simulink model "spaceship_sim_sol_Euler"  (R2023b)
settings: Solver=ode45  StartTime=0.0  StopTime=30  RelTol=1e-3  EnableMultiTasking=on
values from neighbouring files (symbols this model uses):
  Ic = diag([ 1/12*m*H^2+1/4*m*R^2 ; 1/12*m*H^2+1/4*m*R^2 ; 1/2*m*R^2 ])    [spaceship_par_sol.m]
  m = 9600    [par.m]    (also in spaceship_par_sol.m = 12055)
  M_RB = [ m*eye(3) , zeros(3) ; zeros(3) , Ic ]    [spaceship_par_sol.m]
libraries: vrlib x3, simulink_extras x2, sharedtransform x1
Description:
  | Plane Take-Off with HUD Text
  | 
  | This model is a variant of the vrtkoff example that shows also how to display
  | signal values as text in the virtual scene and a simple Head-Up Display (HUD).
  | 
  | The text is sent to the virtual world as Simulink(R) string signal, composed from the numeric
  | input values using the format string (see sprintf for more information) and sent
  | to the 'string' field of the corresponding Text node in the world. Individual lines of
  | the MFString field are separated by the newline character in the format string.
  | 
  | The HUD behavior (maintaining constant relative position between the user and the
  | Text node) is achieved by defining a ProximitySensor that senses user position and
  | orientation as it navigates through the scene and routing this information to the translation
  | and rotation of HUD object - in this case a VRML Transform that contains the Text node.
settings Model: Creator=The MathWorks, Inc.  LastModifiedBy=jerome
settings SolverCC: AlgebraicLoopSolver=TrustRegion
settings DataIOCC: LimitDataPoints=on  SaveFormat=Array  SaveOutput=off  SaveTime=off  ReturnWorkspaceOutputs=off  SignalLoggingName=logsOut
settings OptimizationCC: BlockReduction=off  BooleanDataType=off  ExpressionDepthLimit=2147483647  InitFltsAndDblsToZero=on  LifeSpan=inf
settings DebuggingCC: UnderspecifiedInitializationDetection=Classic  MergeDetectMultiDrivingBlocksExec=none  CheckExecutionContextPreStartOutputMsg=on  SignalResolutionControl=TryResolveAllWithWarning  MultiTaskDSMMsg=warning  MultiTaskCondExecSysMsg=none  FcnCallInpInsideContextMsg=warning  UnconnectedInputMsg=warning  UnconnectedOutputMsg=warning  UnconnectedLineMsg=warning  StateNameClashWarn=warning  SymbolicDimsDataTypeCodeGenerationDiagnostic=none  SFUnexpectedBacktrackingDiag=warning  SFNoUnconditionalDefaultTransitionDiag=warning  SFExecutionAtInitializationDiag=none  ArithmeticOperatorsInVariantConditions=warning
settings HardwareCC: ProdBitPerPointer=32  ProdBitPerSizeT=32  ProdBitPerPtrDiffT=32  ProdLargestAtomicFloat=None  ProdIntDivRoundTo=Undefined  ProdEndianess=Unspecified  ProdWordSize=32  ProdHWDeviceType=32-bit Generic  TargetUnknown=on
settings ModelReferenceCC: UpdateModelReferenceTargets=IfOutOfDate  EnableRefExpFcnMdlSchedulingChecks=on  PropagateSignalLabelsOutOfModel=off
settings SFSimCC: SimUseLocalCustomCode=off  CustomCodeUndefinedFunction=UseInterfaceOnly
settings RTWCC: RTWUseLocalCustomCode=off  DLArmComputeVersion=19.05
settings CodeAppCC: StateflowObjectComments=on
settings GRTTargetCC: TargetFcnLib=ansi_tfl_tmw.mat  TargetLangStandard=C89/C90 (ANSI)  CombineOutputUpdateFcns=off  GRTInterface=on
settings ConfigComp: CovMetricSettings=d  CovSaveCumulativeToWorkspaceVar=on  CovSaveSingleToWorkspaceVar=on  CovExternalEMLEnable=off  CovSFcnEnable=off

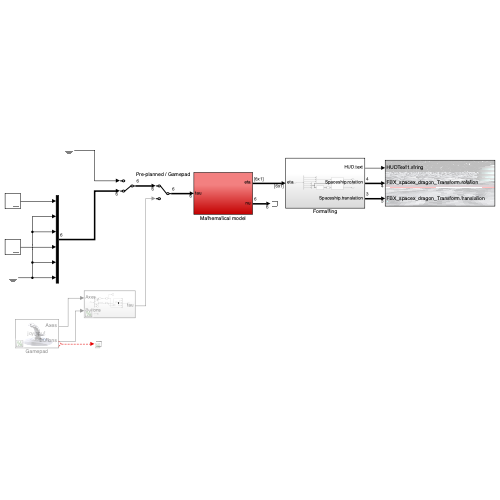
[thumbnail: Simulink's stored preview of the top-level diagram]
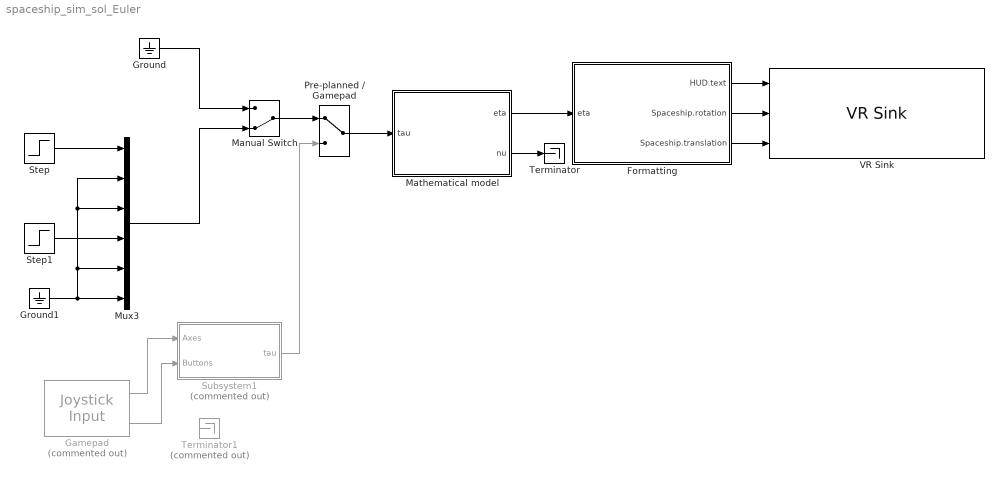
== system spaceship_sim_sol_Euler ==
  Formatting : Subsystem
  Gamepad : vrlib/Joystick Input  Commented=on  joyid=1  adjustports=on  forcefeed=off
  Ground : Ground
  Ground1 : Ground
  Manual Switch : ManualSwitch  CurrentSetting=0
  Mathematical model : Subsystem
  Mux3 : Mux  Inputs=6
  Pre-planned / Gamepad : ManualSwitch
  Step : Step  Before=50000  After=0  SampleTime=0
  Step1 : Step  Before=20000  After=0  SampleTime=0
  Subsystem1 : Subsystem  Commented=on
  Terminator : Terminator
  Terminator1 : Terminator  Commented=on
  VR Sink : vrlib/VR Sink  InstantiateOnLoad=on  SampleTime=0.1  ViewEnable=on  RemoteChange=off  RemoteView=off  FieldsWritten=HUDText1.string.1.-1.1.char#FBX_spacex_dragon_Transform.rotation.4.1.1.double#FBX_spacex_dragon_Transform.translation.3.1.1.double  WorldFileName=spaceship_VR.x3d  WorldDescription=VR Spaceship Dragon  AutoView=off  VideoDimensions=[]  AllowVariableSize=off  FigureProperties="{'Position', 'Name', 'Viewpoint', 'CameraBound', 'CameraDirection', 'CameraPosition', 'CameraUpVector', 'ZoomFactor', 'Antialiasing', 'Headlight', 'Lighting', 'NavPanel', 'Sound', 'StatusBar', 'Stereo3D', 'Stereo3DCameraOffset', 'Stereo3DHIT', 'ToolBar', 'Textures', 'Transparency', 'Triad', 'Wireframe', 'NavZones', 'NavMode', 'NavSpeed', 'CaptureFileFormat', 'CaptureFileName', 'Record2DCompressMethod', 'Record2DCompressQuality', 'Record2D', 'Record2DFileName', 'Record2DFPS'; [5.0000000000000000e+00   1.1600000000000000e+02   5.7600000000000000e+02   3.5000000000000000e+02], 'VR Spaceship Dragon', 'Spaceport', 'on', [0.0000000000000000e+00   0.0000000000000000e+00  -1.0000000000000000e+00], [0.0000000000000000e+00   0.0000000000000000e+00   0.0000000000000000e+00], [0.0000000000000000e+00   1.0000000000000000e+00   0.0000000000000000e+00], [1.0000000000000000e+00], 'on', 'on', 'on', 'halfbar', 'on', 'on', 'off', [1.0000000149011612e-01], [0.0000000000000000e+00], 'on', 'on', 'on', 'none', 'off', 'off', 'fly', 'normal', 'tif', '%f_anim_%n.tif', 'auto', [7.5000000000000000e+01], 'off', '%f_anim_%n.avi', 'auto'}"
  wires:
  Formatting/1(HUD.text) -> VR Sink/1
  Formatting/2(Spaceship.rotation) -> VR Sink/2
  Formatting/3(Spaceship.translation) -> VR Sink/3
  Mathematical model/1(eta) -> Formatting/1(eta)
  Mathematical model/2(nu) -> Terminator/1
  Ground/1 -> Manual Switch/1
  Mux3/1 -> Manual Switch/2
  Ground1/1 -> Mux3/6, Mux3/2, Mux3/3, Mux3/5
  Pre-planned / Gamepad/1 -> Mathematical model/1(tau)
  Manual Switch/1 -> Pre-planned / Gamepad/1
  Gamepad/1 -> Subsystem1/1(Axes)
  Subsystem1/1(tau) -> Pre-planned / Gamepad/2
  Gamepad/2 -> Subsystem1/2(Buttons)
  ? -> Terminator1/1
  Step/1 -> Mux3/1
  Step1/1 -> Mux3/4

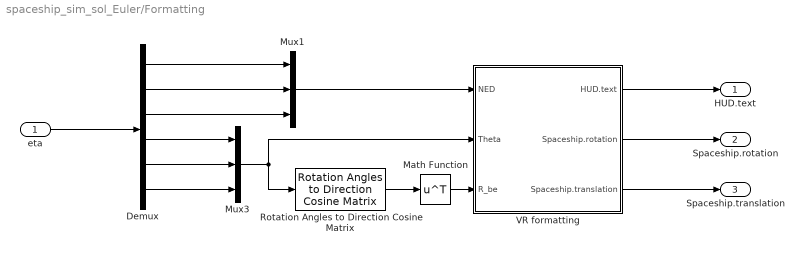
== system spaceship_sim_sol_Euler/Formatting ==
  eta : Inport
  Demux : Demux  Outputs=6
  Math Function : Math  Operator=transpose
  Mux1 : Mux  Inputs=3
  Mux3 : Mux  Inputs=3
  Rotation Angles to Direction Cosine Matrix : sharedtransform/Rotation Angles to Direction Cosine Matrix  rotationOrder=XYZ  aMode=aMode
  VR formatting : Subsystem
  HUD.text : Outport
  Spaceship.rotation : Outport  Port=2
  Spaceship.translation : Outport  Port=3
  wires:
  Demux/2 -> Mux1/2
  Demux/3 -> Mux1/3
  Mux1/1 -> VR formatting/1(NED)
  Demux/5 -> Mux3/2
  eta/1 -> Demux/1
  Demux/4 -> Mux3/1
  Demux/6 -> Mux3/3
  Math Function/1 -> VR formatting/3(R_be)
  Rotation Angles to Direction Cosine Matrix/1 -> Math Function/1
  Demux/1 -> Mux1/1
  VR formatting/1(HUD.text) -> HUD.text/1
  VR formatting/2(Spaceship.rotation) -> Spaceship.rotation/1
  VR formatting/3(Spaceship.translation) -> Spaceship.translation/1
  Mux3/1 -> Rotation Angles to Direction Cosine Matrix/1, VR formatting/2(Theta)

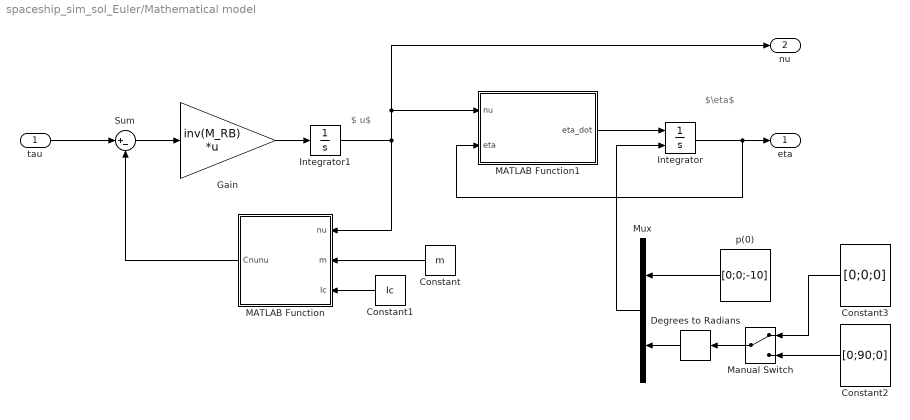
== system spaceship_sim_sol_Euler/Mathematical model ==
  note: $\eta$
  note: $\nu$
  tau : Inport
  Constant : Constant  Value=m
  Constant1 : Constant  Value=Ic  VectorParams1D=off
  Constant2 : Constant  Value=[0;90;0]  VectorParams1D=off
  Constant3 : Constant  Value=[0;0;0]  VectorParams1D=off
  Degrees to Radians : simulink_extras/Transformations/Degrees to Radians
  Gain : Gain  Gain=inv(M_RB)  Multiplication=Matrix(K*u) (u vector)
  Integrator : Integrator  InitialConditionSource=external  InitialCondition=[0;0;-10;0;pi/2;0]
  Integrator1 : Integrator  InitialCondition=[0;0;0;0;0;0]
  MATLAB Function : MATLAB Function  TreatAsAtomicUnit=on
  MATLAB Function1 : MATLAB Function  TreatAsAtomicUnit=on
  Manual Switch : ManualSwitch
  Mux : Mux  Inputs=2
  Sum : Sum  Inputs=|+-
  p(0) : Constant  Value=[0;0;-10]  VectorParams1D=off
  eta : Outport
  nu : Outport  Port=2
  wires:
  Integrator/1 -> eta/1, MATLAB Function1/2(eta)
  Integrator1/1 -> MATLAB Function1/1(nu), nu/1, MATLAB Function/1(nu)
  MATLAB Function1/1(eta_dot) -> Integrator/1
  Constant/1 -> MATLAB Function/2(m)
  Constant1/1 -> MATLAB Function/3(Ic)
  p(0)/1 -> Mux/1
  Degrees to Radians/1 -> Mux/2
  Mux/1 -> Integrator/2
  Gain/1 -> Integrator1/1
  tau/1 -> Sum/1
  Sum/1 -> Gain/1
  MATLAB Function/1(Cnunu) -> Sum/2
  Manual Switch/1 -> Degrees to Radians/1
  Constant2/1 -> Manual Switch/2
  Constant3/1 -> Manual Switch/1

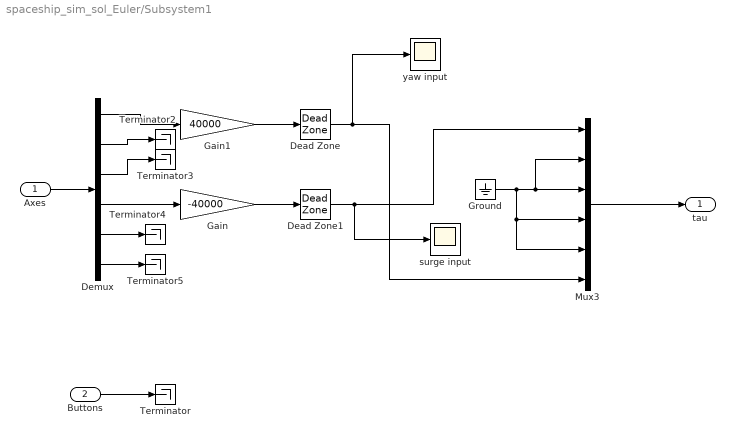
== system spaceship_sim_sol_Euler/Subsystem1 ==
  Axes : Inport
  Buttons : Inport  Port=2
  Dead Zone : DeadZone  LowerValue=-200  UpperValue=200
  Dead Zone1 : DeadZone  LowerValue=-200  UpperValue=200
  Demux : Demux  Outputs=6
  Gain : Gain  Gain=-40000
  Gain1 : Gain  Gain=40000
  Ground : Ground
  Mux3 : Mux  Inputs=6
  Terminator{,2..5} (5 alike) : Terminator
  surge input : Scope
  yaw input : Scope
  tau : Outport
  wires:
  Mux3/1 -> tau/1
  Buttons/1 -> Terminator/1
  Axes/1 -> Demux/1
  Demux/2 -> Terminator2/1
  Demux/3 -> Terminator3/1
  Demux/5 -> Terminator4/1
  Demux/6 -> Terminator5/1
  Ground/1 -> Mux3/3, Mux3/2, Mux3/4, Mux3/5
  Demux/1 -> Gain1/1
  Gain1/1 -> Dead Zone/1
  Dead Zone/1 -> Mux3/6, yaw input/1
  Demux/4 -> Gain/1
  Gain/1 -> Dead Zone1/1
  Dead Zone1/1 -> surge input/1, Mux3/1

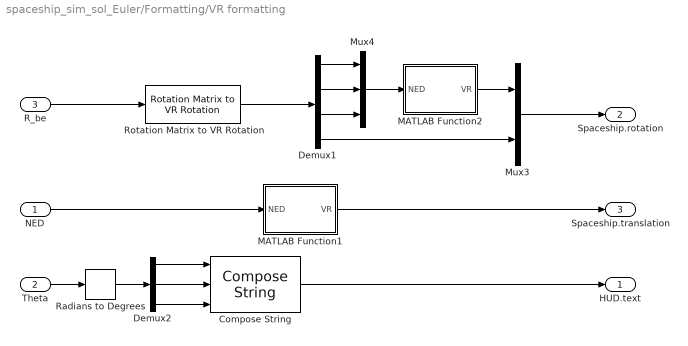
== system spaceship_sim_sol_Euler/Formatting/VR formatting ==
  NED : Inport
  Theta : Inport  Port=2
  R_be : Inport  Port=3
  Compose String : ComposeString  Format="'Roll    : %7.2f deg\\nPitch   : %7.2f deg\\nYaw     : %7.2f deg'"
  Demux1 : Demux
  Demux2 : Demux  Outputs=3
  MATLAB Function1 : MATLAB Function  TreatAsAtomicUnit=on
  MATLAB Function2 : MATLAB Function  TreatAsAtomicUnit=on
  Mux3 : Mux  Inputs=2
  Mux4 : Mux  Inputs=3
  Radians to Degrees : simulink_extras/Transformations/Radians to Degrees
  Rotation Matrix to VR Rotation : vrlib/Utilities/Rotation Matrix to VR Rotation  maxzero=1e-12
  HUD.text : Outport
  Spaceship.rotation : Outport  Port=2
  Spaceship.translation : Outport  Port=3
  wires:
  Rotation Matrix to VR Rotation/1 -> Demux1/1
  Mux3/1 -> Spaceship.rotation/1
  MATLAB Function2/1(VR) -> Mux3/1
  Mux4/1 -> MATLAB Function2/1(NED)
  Demux1/3 -> Mux4/3
  Demux1/1 -> Mux4/1
  Demux1/2 -> Mux4/2
  Demux1/4 -> Mux3/2
  NED/1 -> MATLAB Function1/1(NED)
  MATLAB Function1/1(VR) -> Spaceship.translation/1
  Demux2/1 -> Compose String/1
  Demux2/2 -> Compose String/2
  Demux2/3 -> Compose String/3
  Compose String/1 -> HUD.text/1
  Theta/1 -> Radians to Degrees/1
  R_be/1 -> Rotation Matrix to VR Rotation/1
  Radians to Degrees/1 -> Demux2/1

== matlab function spaceship_sim_sol_Euler/Mathematical model/MATLAB Function1 ==
  data: nu input; eta input; eta_dot output
function eta_dot = J_Theta(nu,eta)

% Euler angle extraction
phi = eta(4);
theta = eta(5);
psi = eta(6);

R_xphi = [ 1 0 0 ; 0 cos(phi) -sin(phi) ; 0 sin(phi) cos(phi) ];
R_ytheta = [ cos(theta) 0 sin(theta) ; 0 1 0 ; -sin(theta) 0 cos(theta) ];
R_zpsi = [ cos(psi) -sin(psi) 0 ; sin(psi) cos(psi) 0 ; 0 0 1 ];

% rotation matrix
R_be = R_zpsi * R_ytheta * R_xphi;

% angular velocity transformation
T_Theta = [ 1 sin(phi)*tan(theta) cos(phi)*tan(theta) ; 0 cos(phi) -sin(phi) ; 0 sin(phi)/cos(theta) cos(phi)/cos(theta) ];

J_Theta = [ R_be , zeros(3) ; zeros(3) , T_Theta ];

eta_dot = J_Theta*nu;

== matlab function spaceship_sim_sol_Euler/Formatting/VR formatting/MATLAB Function1 ==
  data: NED input; VR output
function VR = NED2VR(NED)

x = NED(1); % north
y = NED(2); % east 
z = NED(3); % down

VR = [ -y ; -z ; x ];

== matlab function spaceship_sim_sol_Euler/Formatting/VR formatting/MATLAB Function2 ==
  data: NED input; VR output
function VR = NED2VR(NED)

x = NED(1); % north
y = NED(2); % east 
z = NED(3); % down

VR = [ -y ; -z ; x ];

== matlab function spaceship_sim_sol_Euler/Mathematical model/MATLAB Function ==
  data: nu input; Cnunu output; m input; Ic input
function Cnunu = fcn(nu,m,Ic)

v = nu(1:3);  % linear velocities (expressed in the body frame)
omega = nu(4:6); % angular velocities (expressed in the body frame)


Cnunu = [ cross(omega,m*v) ; -cross(Ic*omega,omega) ];
